simulink model "M5_2301EE20_exp07_120degreeModeusingSine"  (R2024b)
settings: Solver=VariableStepAuto  StartTime=0.0  StopTime=0.04  RelTol=1e-3
libraries: spsIGBTLib x6, spsDCVoltageSourceLib x1, spsThreePhaseParallelRLCLoadLib x1, spsThreePhaseVIMeasurementLib x1, sps_lib x1
settings Model: Creator=prasa  LastModifiedBy=prasa

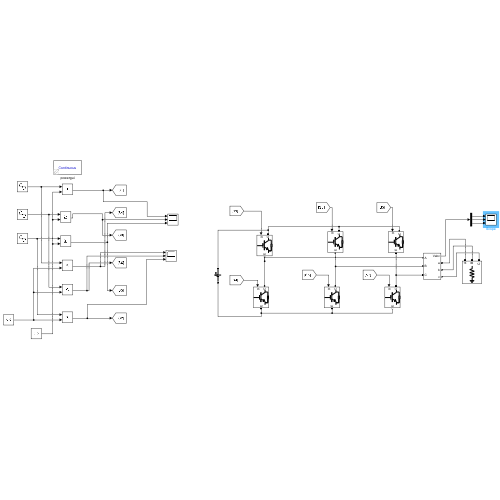
[thumbnail: Simulink's stored preview of the top-level diagram]
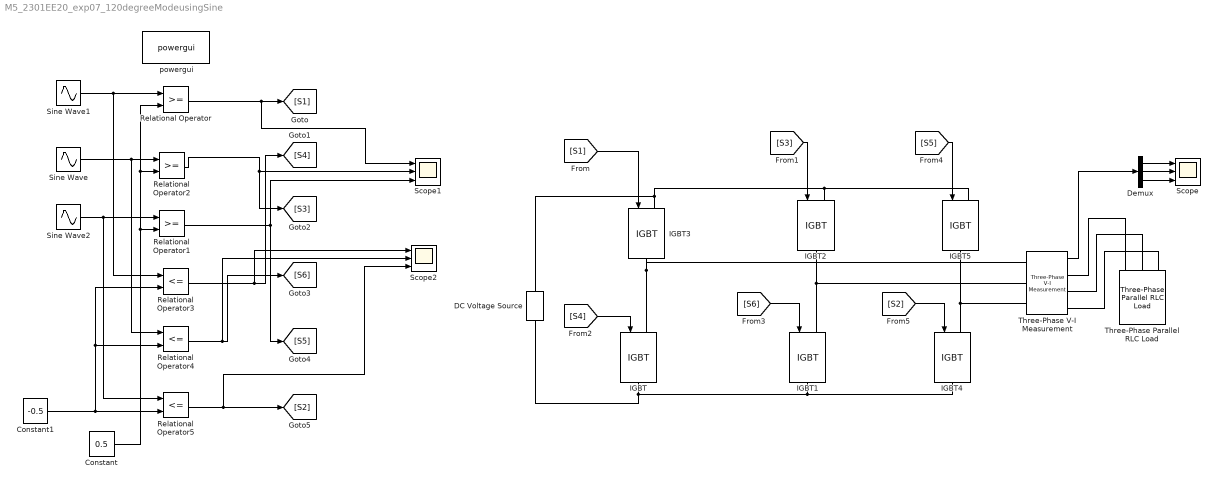
== system M5_2301EE20_exp07_120degreeModeusingSine ==
  Constant : Constant  Value=0.5
  Constant1 : Constant  Value=-0.5
  DC Voltage Source : spsDCVoltageSourceLib/DC Voltage Source  Amplitude=400  Measurements=None
  Demux : Demux  Outputs=3
  IGBT{,1..5} (6 alike) : spsIGBTLib/IGBT  Ron=0.001  Lon=0  Vf=1  Tf=1e-6  Tt=2e-6  IC=0  Rs=1e5  Cs=inf  Measurements=off
  Relational Operator : RelationalOperator  OutDataTypeStr=boolean  RndMeth=Simplest  InputSameDT=off
  Relational Operator1 : RelationalOperator  OutDataTypeStr=boolean  RndMeth=Simplest  InputSameDT=off
  Relational Operator2 : RelationalOperator  OutDataTypeStr=boolean  RndMeth=Simplest  InputSameDT=off
  Relational Operator3 : RelationalOperator  Operator=<=  OutDataTypeStr=boolean  RndMeth=Simplest  InputSameDT=off
  Relational Operator4 : RelationalOperator  Operator=<=  OutDataTypeStr=boolean  RndMeth=Simplest  InputSameDT=off
  Relational Operator5 : RelationalOperator  Operator=<=  OutDataTypeStr=boolean  RndMeth=Simplest  InputSameDT=off
  Scope : Scope  NumInputPorts=3
  Scope1 : Scope  NumInputPorts=3
  Scope2 : Scope  NumInputPorts=3
  Sine Wave : Sin  Frequency=2*pi*50  Phase=-2*pi/3  SampleTime=0
  Sine Wave1 : Sin  Frequency=2*pi*50  SampleTime=0
  Sine Wave2 : Sin  Frequency=2*pi*50  Phase=-4*pi/3  SampleTime=0
  Three-Phase Parallel RLC Load : spsThreePhaseParallelRLCLoadLib/Three-Phase Parallel RLC Load  LConnTagsString=A|B|C  Configuration=Y (grounded)  NominalVoltage=500  Vabc=[1e3 1e3 1e3]  Vabcp=[1e3 1e3 1e3]  NominalFrequency=50  UnbalancedPower=off  ActivePower=10e3  InductivePower=0  CapacitivePower=0  Pabc=[10e3 9e3 11e3]  QLabc=[100 90 110]  QCabc=[100 90 110]  Pabcp=[10e3 9e3 11e3]  QLabcp=[100 90 110]  QCabcp=[100 90 110]  Measurements=None  LoadType=constant Z
  Three-Phase V-I Measurement : spsThreePhaseVIMeasurementLib/Three-Phase V-I Measurement  VoltageMeasurement=phase-to-ground  SetLabelV=off  LabelV=Vabc  Vpu=off  VpuLL=off  CurrentMeasurement=no  SetLabelI=off  LabelI=Iabc  Ipu=off  Pbase=100e6  Vbase=500e3  OutputType=Complex  PhasorSimulation=off  PSBequivalent=0
  powergui : sps_lib/powergui  Priority=1  SimulationMode=Continuous  SampleTime=50e-6  frequency=60  Iterations=50  frequencyindice=0  Pbase=100e6  ErrMax=1e-4  UnitsV=kV  UnitsW=MW  buscounter=0  FunctionMessages=off  echomessages=off  EnableUseOfTLC=off  CurrentSourceSwitches=off  DisableSnubberDevices=off  DisableRonSwitches=off  DisableVfSwitches=off  DisplayEquations=off  AutomaticDiscreteSolvers=off  SolverType=Tustin/Backward Euler (TBE)  Interpol=off  ExternalGateDelay=off  methode=off  Ts=100  x0status=blocks  SPID=on  SwTol=0  HookPort=off  NonlinearTolerance=1e-4  nMaxIteration=100  ContinueOnMaxIteration=off  RestoreLinks=warning  ResistiveCurrentMeasurement=off  Frange=[0:2:500]  Ylog=off  Xlog=on  ShowGrid=off  save=off  variable=ZData  structure=0  ZoomFFT=off  StartTime=0.0  cycles=1  DisplayStyle=1  fundamental=60  FreqAxis=off  MaxFrequency=1000  frequencyindicesteady=1  RmsSteady=1  display=off
  wires:
  [S4] -> IGBT/1
  [S6] -> IGBT1/1
  Demux/1 -> Scope/1
  [S1] -> IGBT3/1
  [S3] -> IGBT2/1
  [S2] -> IGBT4/1
  Demux/2 -> Scope/2
  [S5] -> IGBT5/1
  Demux/3 -> Scope/3
  Sine Wave2/1 -> Relational Operator5/1, Relational Operator1/1
  Relational Operator1/1 -> [S5], Scope1/3
  Relational Operator/1 -> Scope1/1, [S1]
  Sine Wave1/1 -> Relational Operator3/1, Relational Operator/1
  Constant/1 -> Relational Operator1/2, Relational Operator2/2, Relational Operator/2
  Sine Wave/1 -> Relational Operator4/1, Relational Operator2/1
  Relational Operator2/1 -> [S3], Scope1/2
  Constant1/1 -> Relational Operator3/2, Relational Operator4/2, Relational Operator5/2
  Relational Operator3/1 -> Scope2/1, [S4]
  Relational Operator4/1 -> Scope2/2, [S6]
  Relational Operator5/1 -> Scope2/3, [S2]
  Three-Phase V-I Measurement/1 -> Demux/1
  connections:
  Three-Phase V-I Measurement/LConn3 -- IGBT4/LConn1 -- IGBT5/RConn1
  DC Voltage Source/LConn1 -- IGBT1/RConn1 -- IGBT4/RConn1 -- IGBT/RConn1
  Three-Phase V-I Measurement/LConn2 -- IGBT2/RConn1 -- IGBT1/LConn1
  DC Voltage Source/RConn1 -- IGBT2/LConn1 -- IGBT5/LConn1 -- IGBT3/LConn1
  Three-Phase V-I Measurement/LConn1 -- IGBT3/RConn1 -- IGBT/LConn1
  Three-Phase V-I Measurement/RConn2 -- Three-Phase Parallel RLC Load/LConn2
  Three-Phase V-I Measurement/RConn3 -- Three-Phase Parallel RLC Load/LConn3
  Three-Phase V-I Measurement/RConn1 -- Three-Phase Parallel RLC Load/LConn1
